simulink model "sim_discrete_planar_7dof"  (R2023b)
settings: Solver=VariableStepAuto  StartTime=0.0  StopTime=T_sim  FixedStep=param_global.Ta  RelTol=1e-3
InitFcn:
  | parameters_7dof;
undefined symbols (not defined in the file): fx, fy, fz, init_bus_param, param_global, param_robot, param_vis, path_param, q_0, q_0_p, tau_x, tau_y, tau_z
(part 2 of 2)

== matlab function sim_discrete_planar_7dof/Simulation models/controller/path snap controller new fun/path_snap_core ==
  settings: updateMethod=DISCRETE  sampleTime=param_global.Ta
  data: robot_model input Bus: robot_model; tau_iiwa output; q_d_lin_p output; q_d_pp output; path_snap_mode input; motion_enabled input; color_bus output Bus: color_bus; init_bus_param parameter; path_param parameter; param_global parameter; param_robot parameter; debug_snap_data output Bus: debug_snap_data_bus
function [tau_iiwa, q_d_lin_p, q_d_pp, color_bus, debug_snap_data]= path_snap_core(robot_model, path_snap_mode, motion_enabled, init_bus_param, path_param, param_global, param_robot)

    reset_path = 0;
    theta_star_arr = calc_theta_star(robot_model, reset_path, path_param, param_global);
    transport_frame = calc_transport_frame(theta_star_arr, init_bus_param, param_global, path_param);
    path_data = calc_path_data(robot_model, theta_star_arr, transport_frame, init_bus_param, param_global, path_param);

    %% Controller Core

    debug_snap_data = init_bus_param.init_debug_snap_data_bus;
    color_bus = init_bus_param.init_color_bus;
    
    % Desired Velocity of Axis (integrator)
    persistent q_d_lin_p_;
    
    % timer for integrator initalization: if integrator is enabled directly
    % after motion enable, windup will happen because axis are not ready to
    % move sometimes
    persistent timer_init;
    
    % da set_color nur einen Abtastschritt lang 1 sein soll (farbe wird
    % übernommen) und im nächsten Abtastschritt auf 0 gesetzt werden soll, wird
    % persistent Variable benötigt.
    persistent old_color_
    
    if(isempty(q_d_lin_p_)|| ~motion_enabled)
        q_d_lin_p_=zeros(2,1); % reset of Integrator
    end
    
    if(isempty(timer_init)|| ~motion_enabled)
        timer_init = 0;
    end
    
    if( isempty(old_color_) )
        old_color_ = 0;
    end
    
    integrator_inittime = path_param.integrator_inittime;
    
    %% INIT path_param
    q_n = path_param.q_n;
    
    c = path_param.c;
    c_r = path_param.c_r;
    
    d_0 = path_param.d_0;
    d_r0 = path_param.d_r0;
    
    c_dam = path_param.c_dam;
    c_r_dam = path_param.c_r_dam;
    
    Md = path_param.Md;
    Md_r = path_param.Md_r;
    Mdr_osnap = path_param.Mdr_osnap;

    theta_a = path_param.theta_a;
    
    Kd_tang_offpath = path_param.Kd_tang_offpath;
    Kd = path_param.Kd;
    Kd_r = path_param.Kd_r;
    Kdr_osnap = path_param.Kdr_osnap;
    
    Dd_tang_offpath = path_param.Dd_tang_offpath;
    Dd = path_param.Dd;
    Dd_r = path_param.Dd_r;
    Ddr_osnap = path_param.Ddr_osnap;
    
    K_n = path_param.K_n;

    % für gradientenbasierten nullspace controller
    K_n_grad = path_param.K_n_grad;
  
    D_n = path_param.D_n;
    D_dam_t = path_param.D_dam_t;
    D_dam_r = path_param.D_dam_r;
    
    %F_ht = path_param.F_ht;
    F_hr = path_param.F_hr;
    
    N_path = param_global.N_path;
    
    d_mu_0 = path_param.d_mu_0;
    d_mur_0 = path_param.d_mur_0;
    
    xi_1_min = path_param.xi_1_min;
    xi_1_max = path_param.xi_1_max;
    
    xi_d_arr = path_param.xi_d;
    xi_dp_arr = path_param.xi_d_p;
    xi_dpp_arr = path_param.xi_d_pp;
    
    n_phi = path_param.n_phi;
    n_theta = path_param.n_theta;
    n_psi = path_param.n_psi;

    %% extract path_data
    
    %theta_star_arr = path_data.theta_star;
    theta_star_p_arr = path_data.theta_star_p;
    theta_star_pp_arr = path_data.theta_star_pp;
    
    xi_arr = path_data.xi;
    xi_p_arr = path_data.xi_p;
    
    J_hat_arr = path_data.J_hat;
    J_hat_p_arr = path_data.J_hat_p;
    
    %% extract parameters from structs
    M = robot_model.M;      % inertia matrix
    Mqq = M(3:9,3:9);       % inertia marix iiwa
    Mqr = M(3:9,1:2);       % intertia matrix iiwa to xy axis
    C = robot_model.C;      % coriolis matrix
    Cqq = C(3:9,3:9);       % coriolis matrix iiwa
    Cqr = C(3:9,1:2);       % coriolis matrix iiwa to xy axis
    
    q = robot_model.q;
    q_p = robot_model.q_p;
    g = robot_model.g;
    g_iiwa = g(3:9);
    R_e = robot_model.H(1:3,1:3);
    yt = robot_model.H(1:3,4);
    Jt_p = robot_model.J_p(1:3,:);
    Jt = robot_model.J(1:3,:);
    J_p = robot_model.J_p;
    J = robot_model.J;
    J_inv = pinv(J);
    J_iiwa = robot_model.J_iiwa;
    J_iiwa_inv = pinv(J_iiwa);
    J_part_iiwa = robot_model.J_part_iiwa;
    
    y_p = J*q_p;
    yt_p = y_p(1:3);
    omega = y_p(4:6);
    
    % TODO vectorize, effizienter und übersichtlicher machen
    v_t = zeros(3, N_path);
    d = zeros(N_path,1);
    mu_vec = zeros(N_path,1);
    err_xi = zeros(3,N_path);
    
    switch path_snap_mode
        case 4
            %% ORIENTATION SNAP          
                orientation_array = get_all_orientations(n_phi, n_theta, n_psi);
                [~,~, n_orient] = size(orientation_array);
                err_eps = zeros(3,n_orient);
                
                % TODO vectorize
                % initialize vars
                v_omega = zeros(3, n_orient);
                d_r = zeros(n_orient, 1);
                mu_r_vec = zeros(n_orient, 1);
    
                for i = 1:n_orient
                    % calculate expected acceleration
                    R_sigma = orientation_array(:,:,i);
                    rot_err = compact( quaternion(R_sigma * R_e', 'rotmat','frame'))';
                    %rot_err = rotation2quaternion(R_sigma' * R_e); % achtung auf Vorzeichen bei rotationsfehler!
                    epsilon = rot_err(2:4);
                    err_eps(:,i) = epsilon;
                    
                    % derivative of orientation is 0 (nur bei geradelinigen
                    % Pfaden!)
                    omega_d = zeros(3,1);
                    omega_p_d = zeros(3,1);
    
                    % calculate distances
                    d_r(i) = vecnorm(epsilon);
    
                    % calculate weighting factors
                    mu_r_vec(i) = 1 - 1 / (1 + exp(-2*c_r * (d_r(i)/d_r0 - 1) ));
    
                    % angular velocity due to the frames motion
                    v_omega(:,i) = omega_p_d + Mdr_osnap \ (-Ddr_osnap * (omega - omega_d) - Kdr_osnap * epsilon);
                end
                
                mu_r_vec_old = mu_r_vec;
                mu_vec_old = mu_vec;%=0
                
                % weighted error for plotting
                err_eps_weighted = err_eps * mu_r_vec;
                err_xi_weighted = zeros(3,1);
        case 3
            %% PATH SNAP
            v_omega = zeros(3, N_path);
            mu_r_vec = zeros(N_path,1);
            err_eps = zeros(3,N_path);

            for i = 1:1:N_path
                %[sigma, ~, ~, ~] = get_path_t_functions(i);
                %[sigma_r, dsigma_r, ddsigma_r, ~] = get_path_r_functions(i);
                
                theta_star = theta_star_arr(i);
                theta_star_p = theta_star_p_arr(i);
                theta_star_pp = theta_star_pp_arr(i);
            
                xi_d = xi_d_arr(:,i);
                xi_dp = xi_dp_arr(:,i);
                xi_dpp = xi_dpp_arr(:,i);
            
                xi = xi_arr(:,i);
                xi_p = xi_p_arr(:,i);
            
                J_hat = J_hat_arr(:,:,i);
                J_hat_p = J_hat_p_arr(:,:,i);
            
                %% translation
            
                % calculate the desired acceleration in each system
                %xi_1_isoffpath = double(xi(1) < xi_1_min || xi(1) > xi_1_max);
                if(xi(1) < 0) %(xi(1) < xi_1_min)
                    k0 = Kd(1,1);
                    d0 = Dd(1,1);
                    ka = Kd_tang_offpath;
                    da = Dd_tang_offpath;
                    Kd(1,1) = ka * (theta_star < -theta_a) + (k0 - (ka - k0)/theta_a * theta_star) .* (-theta_a <= theta_star) .* (theta_star < 0);
                    Dd(1,1) = da * (theta_star < -theta_a) + (d0 - (da - d0)/theta_a * theta_star) .* (-theta_a <= theta_star) .* (theta_star < 0);
                    xi_d(1) = xi_1_min(i); %Damit Pfad tangential nicht verlassen werden kann
                elseif(xi(1) > xi_1_max(i))%(xi(1) > xi_1_max)
                    k0 = Kd(1,1);
                    d0 = Dd(1,1);
                    ka = Kd_tang_offpath;
                    da = Dd_tang_offpath;
                    Kd(1,1) = (k0 + (ka - k0)/theta_a * (theta_star-1)) .* (1<theta_star) .* (theta_star < 1+theta_a) + ka * (1+theta_a <= theta_star);
                    Dd(1,1) = (d0 + (da - d0)/theta_a * (theta_star-1)) .* (1<theta_star) .* (theta_star < 1+theta_a) + da * (1+theta_a <= theta_star);
                    xi_d(1) = xi_1_max(i); %Damit Pfad tangential nicht verlassen werden kann
                else
                    xi_d(1) = xi(1); % xi kann entlang des pfads beliebig sein
                end
                v_i = xi_dpp + Md \ ( - Dd * (xi_p - xi_dp) - Kd * (xi - xi_d)); %(4.1)
                err_xi(:,i) = xi - xi_d; % xi_tilde
                
                % calculate the same in base system
                J_xi = J_hat(1:3,:);
                J_xi_inv = pinv(J_xi);
                J_xi_p = J_hat_p(1:3,:);
                v_t(:,i) = (Jt_p*q_p + Jt * J_xi_inv * (v_i - J_xi_p*q_p));
            
                % calculate distances
                [sigma, ~, ~, ~] = eval_path_t(theta_star, i, path_param);
                sigma_val = sigma';

                d(i) = vecnorm( sigma_val - yt );
            
                % calculate weighting factors
                mu_vec(i) = 1 - 1 / (1 + exp(-2*c * (d(i) / d_0 - 1) )); 
            
                %% orientation
            
                [sigma_r_val, dsigma_r_val, ddsigma_r_val, ~] = eval_path_r(theta_star, i, path_param);
            
                rot_err = compact( quaternion(sigma_r_val * R_e', 'rotmat','frame'))';
                %rot_err = rotation2quaternion(sigma_r_val' * R_e); % achtung auf Vorzeichen bei rotationsfehler!
                epsilon = rot_err(2:4);
                err_eps(:,i) = epsilon;

                % Wegen Invarianzeigenschaft muss omega_d_p und omega_d
                % aus theta_star_p und theta_star_pp berechnet werden
                sigma_r_val_p  = dsigma_r_val  * theta_star_p;
                sigma_r_val_pp = ddsigma_r_val * theta_star_p^2 + dsigma_r_val * theta_star_pp;

                omega_d_skew   = sigma_r_val_p  * sigma_r_val';
                omega_p_d_skew = sigma_r_val_pp * sigma_r_val' + sigma_r_val_p * sigma_r_val_p';

                omega_d = unskew(omega_d_skew);
                omega_p_d = unskew(omega_p_d_skew);
                                    
                % angular velocity due to the frames motion
                v_omega(:,i) = omega_p_d + Md_r \ (-Dd_r * (omega - omega_d) - Kd_r * epsilon);
                
                % mu_r can only be nonzero, if mu is non zero -> only on
                % the active path + it is also weighted with a distance
                % factor; altough the distance value can be larger than the
                % one for the orientation snap
                mu_r_vec(i) = 1 * (1-1/( 1+exp(-2*c_r* ( vecnorm(epsilon)/d_r0 - 1) ) ));
            end
            %debug
            mu_r_vec_old = mu_r_vec;
            mu_vec_old = mu_vec;
            
            % take the minimum of translation and rotation
            mu_vec = min(mu_vec, mu_r_vec);
            %mu_vec = 1/2*(mu_vec + mu_r_vec);
            mu_r_vec = mu_vec;
            
            % weighted error for plotting
            err_eps_weighted = err_eps * mu_r_vec;
            err_xi_weighted = err_xi * mu_vec;
        otherwise
            err_eps = zeros(3, N_path);
            v_omega = zeros(3, N_path);
            mu_r_vec = zeros(N_path,1);
    
            mu_r_vec_old = mu_r_vec;
            mu_vec_old = mu_vec;%=0
    
            err_eps_weighted = err_eps * mu_r_vec;
            err_xi_weighted = err_xi * mu_vec;
    end
    
    %% damping
    mu = sum(mu_vec);
    mu_r = sum(mu_r_vec);
    
    nu =    1-1/( 1+exp(-2*c_dam* ( mu/d_mu_0 - 1) ) );
    nu_r =  1-1/( 1+exp(-2*c_r_dam*(mu_r/d_mur_0 - 1)));
    
    v_dam = -nu * D_dam_t * yt_p;
    v_dam_r = -nu_r * D_dam_r * omega;
    
    
    %% nullspace control
    % %% Pritzi nullspace control V0 %%
    % NL spring
    f_kn = nl_spring_force(q, path_param, param_robot);

    % Only one spring active (bad idea):
    %[f_kn_max, f_kn_max_ind] = max(f_kn);
    %f_kn = zeros(size(f_kn));
    %f_kn(f_kn_max_ind) = f_kn_max;
    
    % Joint derivatives for nullspace controller
	m_iiwa = sqrt(det(J_iiwa*J_iiwa'));
	J_part_prod = reshape(J_part_iiwa, 6,7,7).*repmat(J_iiwa_inv', 1, 1, 7);
	m_iiwa_diff = m_iiwa*reshape(sum(J_part_prod, [1 2]), 7,1);
    %m_iiwa_normed = m_iiwa_diff/(norm(m_iiwa_diff, 2));

    % %% alternative: gradient based nullspace V1 %%
    %v_n = (-D_n * q_p - K_n * (q - q_n) + f_kn);
    %v_n = K_n_grad*[0;0;m_iiwa_diff] - D_n*q_p; %(3.57a) TimBoye
    v_n = K_n_grad*[0;0;m_iiwa_diff] - D_n*q_p - K_n * (q - q_n) + f_kn; %(3.57a) TimBoye & Pritzi
    %v_n = K_n_grad*[0;0;m_iiwa_normed] - D_n*q_p - K_n * (q - q_n) + f_kn; %(3.57a) TimBoye & Pritzi
    
    v_nullspace = (eye(9) - J_inv*J) * v_n;
    
    %% torque feedback
    v = zeros(6,1);
    v_t_weighted = v_t * mu_vec;
    v_omega_weighted = v_omega * mu_r_vec;
    
    v(1:3) = v_t_weighted + v_dam;
    v(4:6) = v_omega_weighted + v_dam_r;
    
    % add threshold to ensure F_h is never exceeded -> especially for
    % combined system
    f_r = vecnorm(Md_r * v(4:6));
    if f_r > F_hr
        v(4:6) = v(4:6) / f_r * F_hr;
    end
    
    % feedback (4.13)
    n_iiwa = [Cqr,Cqq]*q_p + g_iiwa; %n = C*q_p + g;
    qpp_temp = J_inv*(v - J_p * q_p); % = v_taskspace
    
    %tau_iiwa = n_iiwa + [Mqr,Mqq]*qpp_temp + tau_n_iiwa;
    tau_iiwa = n_iiwa + [Mqr,Mqq]*(qpp_temp + v_nullspace);
    
    %tau_n = M * v_nullspace; %(3.41) Pritzi
    %tau_n_iiwa = [Mqr,Mqq] * v_nullspace; %(3.41) Pritzi   
    
    %% Linearachsen
    
    % gewünschte Gelenksbeschleunigung
    % von M*qpp + C*qp + g = M*qpp + n = tau
    % qpp = M^(-1) * (tau-n) = M^(-1) * (n + M*qpp_temp + tau_n - n)
    %     = M^(-1) * (M*qpp_temp + tau_n) = qpp_temp + M^(-1)*tau_n
    if(motion_enabled == 1) % sonst rechnet luenberger es reverse damit aus
        q_d_pp = qpp_temp + v_nullspace;
        %q_d_pp = v_nullspace;
    else
        q_d_pp = zeros(9,1);
    end
    
    % nur Beschleunigung der Linearachsen
    % q_lin_pp = q_d_pp(1:2);
    
    q_d_lin_p = q_d_lin_p_;
    
    % Integration
    if timer_init < integrator_inittime % Integrator erst aktivieren, wenn Init-Zeit verstrichen
        timer_init = timer_init + param_global.Ta;
    else
        q_d_lin_pp = q_d_pp(1:2); % nur Beschleunigung der Linearachsen
        q_d_lin_p_ = q_d_lin_p_ + q_d_lin_pp*param_global.Ta; %(3.35) TimBoye%
    end
    
    %% set color
    if(mu_r > 0.5 && mu > 0.5)
        color = 7; % 7 -> both locked: green red blue
    elseif(mu_r > 0.5)
        color = 3; % 3 -> orientation locked: green red
    elseif(mu > 0.5)
        color = 5; % 5 -> translation locked: greenblue
    else
        color = 1; % free :green
    end
    
    if color ~= old_color_
        set_color = 1;
    else
        set_color = 0;
    end
    
    color_bus.color = color;
    color_bus.set_color = set_color;
    
    old_color_ = color;
    
    % debug
    mu_r = sum(mu_r_vec_old);
    mu = sum(mu_vec_old);
    
    %% set Debug Data (comment out and delete output for more performance)
    debug_snap_data.v_dam=v_dam;
    debug_snap_data.v_dam_r=v_dam_r;
    debug_snap_data.v_n=v_n;
    debug_snap_data.v_t_weighted=v_t_weighted;
    debug_snap_data.v_omega_weighted=v_omega_weighted;
    debug_snap_data.mu=mu;
    debug_snap_data.mu_r=mu_r;
    debug_snap_data.err_xi_weighted=err_xi_weighted;
    debug_snap_data.err_eps_weighted=err_eps_weighted;
    debug_snap_data.nu=nu;
    debug_snap_data.nu_r=nu_r;
    debug_snap_data.theta_star = theta_star_arr;
    %xx_xi_pp_omega_p = J_hat*q_d_pp + J_hat_p*q_p; % = [xi_pp, omega_p]
    % vectorized version of previous command: results in
    % [xi_D1_pp;xi_D2_pp;...xi_DN_Path_pp] \in R^(3xN_path)
    xx_xi_pp_omega_p_arr = reshape((reshape(J_hat_arr, [6*N_path,9])*q_d_pp), [6,N_path]) + reshape((reshape(J_hat_p_arr, [6*N_path,9])*q_p), [6,N_path]);
    [~,active_path_index_r] = max(mu_r_vec);
    [~,active_path_index_t] = max(mu_vec);
    debug_snap_data.xi = xi_arr;
    debug_snap_data.xi_p = xi_p_arr;
    debug_snap_data.xi_pp = xx_xi_pp_omega_p_arr(1:3,:); % xi_pp differ for each path
    debug_snap_data.epsilon = err_eps(:,1:N_path); % warning: won't work for orientation snap
    debug_snap_data.omega = omega;
    debug_snap_data.omega_p = xx_xi_pp_omega_p_arr(4:6,1); % omega_p is always the same for each path therefore use first
    
    debug_snap_data.Rot_transport_frame = transport_frame.R; % = [transport_frame.e1 transport_frame.e2 transport_frame.e3] als (3x3xNpath)
    %xi_1_vals = path_param.xi_1_data;
    %N_samp = path_param.xi_1_N_samp;
    %xi1_trapez = xi_1_vals(:,1+round(theta_star*(N_samp-1)));
    %debug_snap_data.xi1_trapez = xi1_trapez;
    debug_snap_data.active_path_index_r = active_path_index_r;
    debug_snap_data.active_path_index_t = active_path_index_t;
end





%%%%%%%%%%%%%%%%%%%%%%%%%%%%%%%%%%%%%%%%%%%%%%%%%%%%%%%%%%%%%%%%%%%%%%%%%%%
%%%%%%%%%%%%%%%%%%%%%%%%%%%%%%%% FUNKTIONEN %%%%%%%%%%%%%%%%%%%%%%%%%%%%%%%
%%%%%%%%%%%%%%%%%%%%%%%%%%%%%%%%%%%%%%%%%%%%%%%%%%%%%%%%%%%%%%%%%%%%%%%%%%%




%%%%%%%%%%%%%%%%%%%%%%%%%%%%%%%%%%%%%%%%%%%%%%%%%%%%%%%%%%%%%%%%%%%%%%%%%%%
%% calc_theta_star %%%%%%%%%%%%%%%%%%%%%%%%%%%%%%%%%%%%%%%%%%%%%%%%%%%%%%%%
%%%%%%%%%%%%%%%%%%%%%%%%%%%%%%%%%%%%%%%%%%%%%%%%%%%%%%%%%%%%%%%%%%%%%%%%%%%
function theta_star = calc_theta_star(robot_model, reset_path, path_param, param_global)

    persistent theta;
    
    epsilon = path_param.epsilon;
    N_path = param_global.N_path;
    %theta_min = path_param.theta_min;
    %theta_max = path_param.theta_max;
    
    % get the position of the endeffector from the model
    yt = robot_model.H(1:3,4);
    
    %% INIT GRID:
    % Die Idee ist, zu Beginn ein grobes Grid von theta Werten zu erstellen und
    % einen groben Startwert für theta_star zu berechnen, damit das Newton
    % Verfahren schneller und stabiler konvergiert.
    %
    % reset_path ist daher dafür da, dass man theta grob initialisiert.
    
    if (isempty(theta)) || reset_path >= 1
        theta = path_param.theta_star_start_vals;
        
        %{
        % settings for the global search grid
        par_min = 0;
        par_max = 1;
        par_nr = 20;
    
        % find the best value of the path parameter on the grid as starting
        % value
        theta_grid = linspace(par_min, par_max, par_nr);
        
        for i = 1:N_path
            %[sigma, ~, ~, ~] = get_path_t_functions(i);
            %sigma_grid_vals = sigma(theta_grid)';
            [sigma_grid, ~, ~, ~] = eval_path_t(theta_grid, i, path_param);
            sigma_grid_vals = sigma_grid';

            e = repmat(yt,1, par_nr) - sigma_grid_vals;
            [~, index] = min( vecnorm(e) );
            theta(i) = theta_grid(index);
        end
        
        %}
    end
    
    %% Berechnen von theta_star
    
    theta_star = theta;
    for i = 1:N_path  
        % as long as derivative is not small enough no minimum is found
        while 1 % sollte eine maximale anzahl an schritten einstellen
            [sigma, dsigma, ddsigma, ~] = eval_path_t(theta_star(i), i, path_param);
            sigma_val = sigma';
            dsigma_val = dsigma';
            ddsigma_val = ddsigma';
        
            d_f = -2 * dsigma_val' * (yt - sigma_val); %(3.9)
            dd_f = -2 * ddsigma_val' * (yt - sigma_val) + 2*norm(dsigma_val)^2; %(3.11)
    
            if(abs(d_f) < epsilon)
                break;
            else
                % Newton step
                if (dd_f ~=0)
                    theta_star(i) = theta_star(i) - d_f / dd_f;
                end
            end
    
    
        end
    end
    
    theta = theta_star;
    
end

%%%%%%%%%%%%%%%%%%%%%%%%%%%%%%%%%%%%%%%%%%%%%%%%%%%%%%%%%%%%%%%%%%%%%%%%%%%
%% calc_transport_frame %%%%%%%%%%%%%%%%%%%%%%%%%%%%%%%%%%%%%%%%%%%%%%%%%%%
%%%%%%%%%%%%%%%%%%%%%%%%%%%%%%%%%%%%%%%%%%%%%%%%%%%%%%%%%%%%%%%%%%%%%%%%%%%
function transport_frame = calc_transport_frame(theta, init_bus_param, param_global, path_param)
    % Diese Funktion berechnet das Transport Frame. Da hier die DAE (5)
    % Bischof2017 (B17) iterativ gelöst wird, wird e2 als persistent Variable
    % gespeichert. Zu Beginn wird e2 initialisiert und N_init iterationen oft
    % iteriert, damit es die DAE erfüllt.
    %
    % Legende:
    % e1 = e_||
    % e2 = e_perp
    % e3 = e_pitchfork
    
    persistent e2_;
    
    N_path = param_global.N_path;
    transport_frame = init_bus_param.init_transport_frame_bus;
    
    %% INIT e2
    if (isempty(e2_))
        e2_ = 1/sqrt(3) * ones(3,N_path); % = e2_0
    end
    
    %% Calculate Transport Frame Vektors and Deviations
    
    for i = 1:1:N_path
        %[~, dsigma, ddsigma, ~] = get_path_t_functions(i);
        %dsigma_val = dsigma(theta(i))';
        %ddsigma_val = ddsigma(theta(i))';
        [~, dsigma, ddsigma, ~] = eval_path_t(theta(i), i, path_param);
        dsigma_val = dsigma';
        ddsigma_val = ddsigma';
    
        % get actual e2 value
        e2 = e2_(:,i);
    
        % Transport Frame Vektors
        e1 = dsigma_val / norm(dsigma_val); % (5) B17
        e2 = (e2 - dot(e1,e2) * e1) / sqrt(1 - (e1' * e2)^2 );
        e3 = cross(e1, e2);
    
        % Transport Frame derivatives
        de1 = 1/norm(dsigma_val) * (ddsigma_val - (e1'*ddsigma_val) * e1);
        de2 = - (de1' * e2) * e1;
        de3 = - (de1' * e3) * e1;
    
        % Write data to transport frame bus
        transport_frame.e1(:,i) = e1;
        transport_frame.e2(:,i) = e2;
        transport_frame.e3(:,i) = e3;
        transport_frame.de1(:,i) = de1;
        transport_frame.de2(:,i) = de2;
        transport_frame.de3(:,i) = de3;
        transport_frame.R(:,:,i) = [e1 e2 e3];
    end
end

%%%%%%%%%%%%%%%%%%%%%%%%%%%%%%%%%%%%%%%%%%%%%%%%%%%%%%%%%%%%%%%%%%%%%%%%%%%
%% calc_path_data %%%%%%%%%%%%%%%%%%%%%%%%%%%%%%%%%%%%%%%%%%%%%%%%%%%%%%%%%
%%%%%%%%%%%%%%%%%%%%%%%%%%%%%%%%%%%%%%%%%%%%%%%%%%%%%%%%%%%%%%%%%%%%%%%%%%%
function path_data = calc_path_data(robot_model, theta_star, transport_frame, init_bus_param, param_global, path_param)
    % Legende
    % e1 = e_||
    % e2 = e_perp
    % e3 = e_pitchfork
    % xi1 = xi_||
    % xi2 = xi_perp
    % xi3 = xi_pitchfork
    
    persistent xi1_;
    persistent xi1p_;
    
    N_path = param_global.N_path;

    if(isempty(xi1_))
        xi1_ = path_param.xi_1_start_vals;
        xi1p_ = zeros(1, N_path);
    end
    
    
    
    path_data = init_bus_param.init_path_data_bus;
    
    %N_samp = path_param.xi_1_N_samp;
    %xi_1_vals = path_param.xi_1_data;
    %theta_min = path_param.theta_min;
    %theta_max = path_param.theta_max;
    %xi_1_min = path_param.xi_1_min;
    %xi_1_max = path_param.xi_1_max;
    %
    %xi1 = zeros(1,N_path);
    
    %% retrieve values
    yt = robot_model.H(1:3, 4); % Aktuelle Endeffektorposition, Vorwärtskinematik
    Jt = robot_model.J(1:3, :); % Translatorische Jacobimatrix (TCP zu Basis)
    Jr = robot_model.J(4:6, :); % Rotatorische Jacobimatrix (TCP zu Basis)
    Jt_p = robot_model.J_p(1:3, :);
    Jr_p = robot_model.J_p(4:6, :);
    
    q_p = robot_model.q_p;
    q_pp = robot_model.q_pp; % ist eig der desired Wert als Näherung für q_pp
    yt_p = Jt * q_p; % d/dt yt
    
    %% extract transport frame
    e1 = transport_frame.e1;
    e2 = transport_frame.e2;
    e3 = transport_frame.e3;
    de1  = transport_frame.de1;
    de2  = transport_frame.de2;
    de3  = transport_frame.de3;
    
    for i = 1:N_path
        %[sigma, dsigma, ddsigma, dddsigma] = get_path_t_functions(i);
        %sigma_val = sigma(theta_star(i))';
        %dsigma_val = dsigma(theta_star(i))';
        %ddsigma_val = ddsigma(theta_star(i))';
        %dddsigma_val = dddsigma(theta_star(i))';

        [sigma, dsigma, ddsigma, dddsigma] = eval_path_t(theta_star(i), i, path_param);
        sigma_val = sigma';
        dsigma_val = dsigma';
        ddsigma_val = ddsigma';
        dddsigma_val = dddsigma';

        dsigma_val_norm = norm(dsigma_val); % = ||d/dt sigma||_2
    
        % 1. calculate theta_p %
    
        d_i = yt - sigma_val; %(4.33), Abweichung zwischen Ist TCP Position yt und sollposition am Pfad sigma(theta_star)
        % d_i ist der kürzeste Abstand vom TCP zum Pfad.
    
        % fragen ob er tangential out of path ist.
        %if(theta_star == theta_min)
        %    xi1(i) = xi_1_min-norm(d_i); %virtuelle gerade damit Pfad tangential nicht verlassen werden kann
        %    %xi1(i) = 0;
        %elseif(theta_star == theta_max)
        %    xi1(i) = xi_1_max+norm(d_i); %virtuelle gerade damit Pfad tangential nicht verlassen werden kann
        %    %xi1(i) = xi_1_vals(i,N_samp);
        %else
        %    xi1(i) = xi_1_vals(i,1+round(theta_star*(N_samp-1)));
        %end
    
        alpha = d_i' * ddsigma_val / norm(dsigma_val)^2; %(3.13)
        m1_alpha = 1-alpha;
    
        beta = 1/m1_alpha; %(3.16)
        theta_star_p = beta * e1(:,i)' * yt_p / norm(dsigma_val);
        
        e1_p = de1(:, i) * theta_star_p;
        e2_p = de2(:, i) * theta_star_p;
        e3_p = de3(:, i) * theta_star_p;
    
        % 2. calculate coordinate values %
    
        xi2 = e2(:,i)' * d_i; %(3.19)
        xi3 = e3(:,i)' * d_i; %(3.20)
    
        xi1p = dsigma_val_norm * theta_star_p; %(3.21)
        xi2p = e2(:,i)' * yt_p; %(3.24)
        xi3p = e3(:,i)' * yt_p; %(3.25)
    
        % 3. calculate jacobian matrices for the new coordinate system %
    
        %alpha_p = d/dt alpha(t) = d/dt u/v = ((d/dt u) * v - u * (d/dt v))/v^2
        % anmk. ich glaube pritzi hatte sich hier verrechnet. unsicher.
        alpha_p = 1/dsigma_val_norm^4 * ( ( (yt_p' - dsigma_val'*theta_star_p)*ddsigma_val + d_i'*dddsigma_val*theta_star_p )*dsigma_val_norm^2 ...
                                          - d_i' * ddsigma_val * 2*dsigma_val_norm*theta_star_p );
        %pritzi old:
        %alpha_p = 1/norm(dsigma_val)^4 * ( ( (yt_p' - dsigma_val'*theta_star_p)*ddsigma_val + (yt' - sigma_val')*dddsigma_val*theta_star_p )*norm(dsigma_val)^2 ...
        %                        -  2 * (yt' - sigma_val') * ddsigma_val * dsigma_val' * ddsigma_val * theta_star_p );
    
        beta_p = alpha_p/m1_alpha^2;
        
        % (3.27) mit J_omega, es ist ja für pfad als auch basis KOS gleich.
        J_hat = [beta * e1(:,i)', zeros(1,3); ...
                e2(:,i)', zeros(1,3); ...
                e3(:,i)', zeros(1,3); ...
                zeros(3), eye(3)] * [Jt; Jr];
        
        % sollte passen, ich sollte das alles aber nochmal nachrechnen.
        J_hat_p = [[beta_p * e1(:,i)' + beta * e1_p'; e2_p'; e3_p'] * Jt + ...
                  [beta * e1(:,i)'; e2(:,i)'; e3(:,i)'] * Jt_p; ...
                  Jr_p];
    
        %
        yt_pp = Jt * q_pp + Jt_p * q_p; % (2.5) abgeleitet
        u = beta * e1(:,i)' * yt_p;
        u_s = (beta_p * e1(:,i)' * yt_p + beta * e1_p' * yt_p + beta * e1(:,i)' * yt_pp)*theta_star_p;
        v = dsigma_val_norm;
        %v_s = theta_star_p * sum(ddsigma_val)/(dsigma_val_norm); % unsicher
        v_s = theta_star_p * e1(:,i)' * ddsigma_val; %Glaube eher das ist korrekt

        theta_star_pp = (u_s * v - u * v_s) / v^2; %(3.17) nach t abgeleitet
    
        % Expliziter Euler:
        % xi1(t+Ta) = theta_star(t+Ta) mit explizitem euler verfahren berechnen:
        % d/dt xi1(t) = xi1_p(t)
        % xi1(t1) - xi1(t0) = int(xi1_p(t), t=t0..t1) ≈ (t1-t0)*xi1_p(t0)
        % mit t1=t+Ta, t0=t folgt
        % xi1(t+Ta) = xi1(t) + Ta*xi1_p(t)
        %
        % wichtig: xi1 entspricht der tangentiellen Länge des Pfades und darf
        % daher nicht mit theta_star verwechselt werden. Z. b. hat ein Pfad,
        % der vom Punkt [0 0 0] zum Punkt [0 0 2] geht die Länge 2, d. h. wenn
        % man zum Zeitpunkt t+Ta am Ende des Pfads ist gilt theta_star=1, xi1=2
    
    
        % zugriff mit path_param.xi_1_data(round(theta*1000)) (update: jetzt
        % nicht mehr)
        
        % heun (ist aber nicht ganz korrekt, eig muesst ich xi1p mit xi1
        % neu berechnen).
        %xi1 = xi1_ + par.Ta*xi1p_;
        %xi1_ = 1/2 * xi1_ + 1/2*(xi1 + par.Ta*xi1p);
        %xi1 = xi1_;
        %xi1p_ = xi1p;

        % expl euler
        xi1_(i) = xi1_(i) + param_global.Ta*xi1p;
        xi1 = xi1_(i);
    
        path_data.theta_star(1, i) = theta_star(i);
        path_data.theta_star_p(1, i) = theta_star_p;
        path_data.theta_star_pp(1, i) = theta_star_pp;
        path_data.xi(1:3, i) = [xi1 xi2 xi3]';
        path_data.xi_p(1:3, i) = [xi1p xi2p xi3p]';
        path_data.J_hat(:,:, i) = J_hat;
        path_data.J_hat_p(:,:, i) = J_hat_p;
    end
end

== matlab function sim_discrete_planar_7dof/Debug Subsystem/MATLAB Function1 ==
  data: debug_data input Bus: debug_data_bus; e_x output; e_y output; e_x_p output; e_y_p output; e_x_pp output; e_y_pp output; x_d_trj input Bus: x_d
function [e_x, e_y, e_x_p, e_y_p, e_x_pp, e_y_pp] = fcn(debug_data, x_d_trj)

p    = debug_data.p;
p_p  = debug_data.p_p;
p_pp = debug_data.p_pp;

p_d    = x_d_trj.p_d;
p_d_p  = x_d_trj.p_d_p;
p_d_pp = x_d_trj.p_d_pp;

e_x    = p_d(1)    - p(1);
e_x_p  = p_d_p(1)  - p_p(1);
e_x_pp = p_d_pp(1) - p_pp(1);

e_y    = p_d(2)    - p(2);
e_y_p  = p_d_p(2)  - p_p(2);
e_y_pp = p_d_pp(2) - p_pp(2);
